simulink model "MotionControl"  (R2023b)
settings: Solver=VariableStepAuto  StartTime=0.0  StopTime=time(end)  RelTol=1e-3
undefined symbols (not defined in the file or in its folder): DiscIntNeverNeededParam
settings Model: Creator=v4pal  LastModifiedBy=v4pal

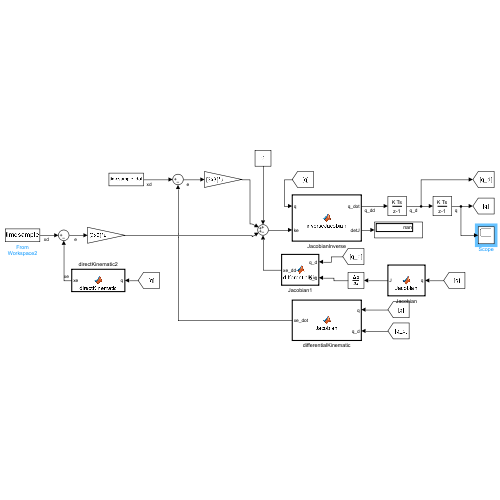
[thumbnail: Simulink's stored preview of the top-level diagram]
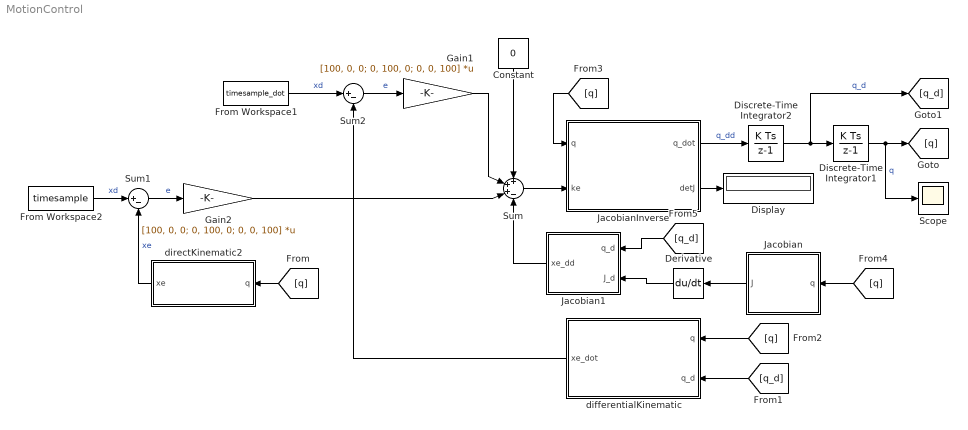
== system MotionControl ==
  Constant : Constant  Value=0
  Derivative : Derivative
  Discrete-Time Integrator1 : DiscreteIntegrator  InitialCondition=[0; pi/4; .25]  SampleTime=0.001  ICPrevOutput=DiscIntNeverNeededParam  ICPrevScaledInput=DiscIntNeverNeededParam
  Discrete-Time Integrator2 : DiscreteIntegrator  InitialCondition=[0; pi/4; .25]  SampleTime=0.001  ICPrevOutput=DiscIntNeverNeededParam  ICPrevScaledInput=DiscIntNeverNeededParam
  Display : Display
  From Workspace1 : FromWorkspace  VariableName=timesample_dot
  From Workspace2 : FromWorkspace  VariableName=timesample
  Gain1 : Gain  Gain=[100, 0, 0; 0, 100, 0; 0, 0, 100]  Multiplication=Matrix(K*u)
  Gain2 : Gain  Gain=[100, 0, 0; 0, 100, 0; 0, 0, 100]  Multiplication=Matrix(K*u)
  Jacobian : MATLAB Function  TreatAsAtomicUnit=on
  Jacobian1 : MATLAB Function  TreatAsAtomicUnit=on
  JacobianInverse : MATLAB Function  TreatAsAtomicUnit=on
  Scope : Scope
  Sum : Sum  Inputs=+++-
  Sum1 : Sum  Inputs=|+-
  Sum2 : Sum  Inputs=|+-
  differentialKinematic : MATLAB Function  TreatAsAtomicUnit=on
  directKinematic2 : MATLAB Function  TreatAsAtomicUnit=on
  wires:
  JacobianInverse/1(q_dot) -> Discrete-Time Integrator2/1  "q_dd"
  Sum1/1 -> Gain2/1  "e"
  From Workspace2/1 -> Sum1/1  "xd"
  directKinematic2/1(xe) -> Sum1/2  "xe"
  Sum/1 -> JacobianInverse/2(ke)
  Gain2/1 -> Sum/3
  Gain1/1 -> Sum/2
  Discrete-Time Integrator2/1 -> [q_d], Discrete-Time Integrator1/1  "q_d"
  Discrete-Time Integrator1/1 -> Scope/1, [q]  "q"
  [q] -> directKinematic2/1(q)
  [q_d] -> differentialKinematic/2(q_d)
  [q] -> differentialKinematic/1(q)
  Sum2/1 -> Gain1/1  "e"
  differentialKinematic/1(xe_dot) -> Sum2/2
  From Workspace1/1 -> Sum2/1  "xd"
  Constant/1 -> Sum/1
  JacobianInverse/2(detJ) -> Display/1
  [q] -> JacobianInverse/1(q)
  Jacobian/1(J) -> Derivative/1
  [q] -> Jacobian/1(q)
  Derivative/1 -> Jacobian1/2(J_d)
  [q_d] -> Jacobian1/1(q_d)
  Jacobian1/1(xe_dd) -> Sum/4

== matlab function MotionControl/differentialKinematic ==
  data: q input; xe_dot output; q_d input
function xe_dot = Jacobian(q, q_d)

    % Init the SCARA manipulator parameters
    a1 = .5; a2 = .5;

    theta1 = q(1,:); theta2 = q(2,:);
    %% Geometric Jacobian Matrix
    J = [-a1*sin(theta1) - a2*sin(theta1 + theta2), - a2*sin(theta1 + theta2), 0, 0;
        a1*cos(theta1) + a2*cos(theta1 + theta2), a2*cos(theta1 + theta2), 0, 0;
        0, 0, -1, 0;
        1, 1, 0, -1;];

    % Vx = Jx1 * qd1 + Jx2 * qd2 +Jx3 * qd3;
    % Vy = Jy1 * qd1 + Jy2 * qd2 +Jy3 * qd3;
    % Vz = Jz1 * qd1 + Jz2 * qd2 +Jz3 * qd3;
    
    J = J(1:3,1:3);

    %% Calculation of xe_dot
    xe_dot = J * q_d;

end

== matlab function MotionControl/directKinematic2 ==
  data: q input; xe output
function xe = directKinematic(q)
    
    %% Init the SCARA manipulator parameters and Joint variables
    a1 = .5; a2 = .5; d0 = 1;
    theta1 = q(1,:); theta2 = q(2,:); d3 = q(3,:);

    %% Forward Kinematics link for the SCARA
    k = [a1*cos(theta1) + a2*cos(theta1 + theta2);
        a1*sin(theta1) + a2*sin(theta1 + theta2);
        d0 - d3;];

    xe = k;

end

== matlab function MotionControl/Jacobian ==
  data: q input; J output
function J = Jacobian(q)

    % Init the SCARA manipulator parameters
    a1 = .5; a2 = .5;

    theta1 = q(1,:); theta2 = q(2,:);

    %% Geometric Jacobian Matrix
    J = [-a1*sin(theta1) - a2*sin(theta1 + theta2), - a2*sin(theta1 + theta2), 0;
        a1*cos(theta1) + a2*cos(theta1 + theta2), a2*cos(theta1 + theta2), 0;
        0, 0, -1];

end

== matlab function MotionControl/Jacobian1 ==
  data: q_d input; xe_dd output; J_d input
function xe_dd = differentialKin(q_d,J_d)
    
    xe_dd = J_d *- q_d;

end

== matlab function MotionControl/JacobianInverse ==
  data: q input; ke input; q_dot output; detJ output
function [q_dot, detJ] = inverseJacobian(q, ke) % q = [theta1; theta2]

    % Init the SCARA manipulator parameters
    a1 = .5; a2 = .5;

    theta1 = q(1,:); theta2 = q(2,:);
    %% Geometric Jacobian Matrix
    J = [-a1*sin(theta1) - a2*sin(theta1 + theta2), - a2*sin(theta1 + theta2), 0, 0;
        a1*cos(theta1) + a2*cos(theta1 + theta2), a2*cos(theta1 + theta2), 0, 0;
        0, 0, -1, 0;
        1, 1, 0, -1;];

    % Vx = Jx1 * qd1 + Jx2 * qd2 +Jx3 * qd3;
    % Vy = Jy1 * qd1 + Jy2 * qd2 +Jy3 * qd3;
    % Vz = Jz1 * qd1 + Jz2 * qd2 +Jz3 * qd3;
    
    J = J(1:3,1:3);
    
    detJ = det(J);
    % Calculate the inverse of the Jacobian matrix
    J_inv = inv(J);

    % Calculate joint velocities
    q_dot = J_inv * ke;

end
